simulink model "test_ENU"  (R2019b)
settings: Solver=VariableStepAuto  StartTime=0.0  StopTime=10.0  RelTol=1e-3
values from neighbouring files (symbols this model uses):
  own_height = 20000    [test_ENU_script.m]
  own_lat = 40    [test_ENU_script.m]
  own_long = 60    [test_ENU_script.m]
  traf_height = 15000    [test_ENU_script.m]
  traf_lat = 40    [test_ENU_script.m]
  traf_long = 60    [test_ENU_script.m]
settings Model: Creator=markwilkinson  LastModifiedBy=markwilkinson

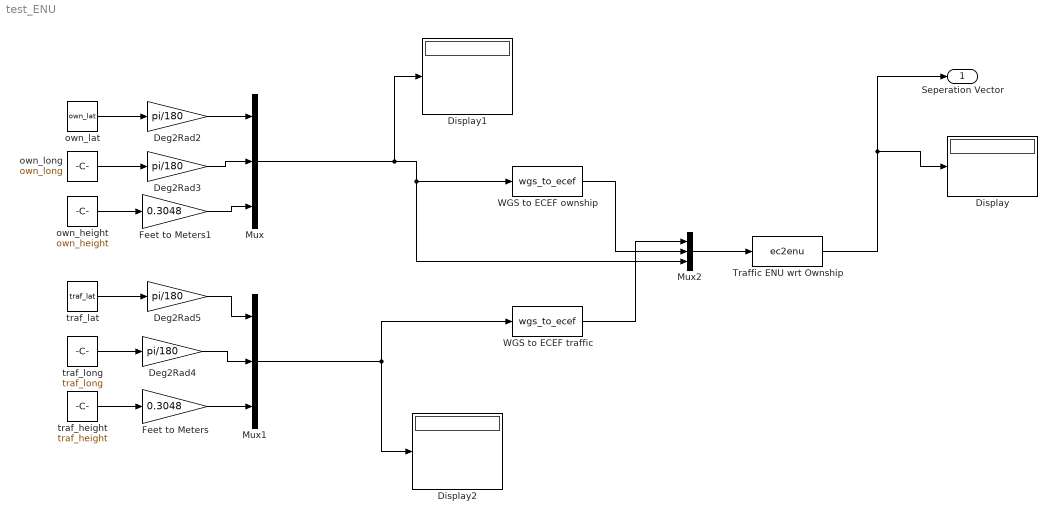
== system test_ENU ==
  Deg2Rad2 : Gain  RequirementInfo="{'other' 'cdf_srd - rev a.xlsx' '@Simulink_requirement_item_11' 'true' 'The system shall apply a gain of (pi/180) to the following inputs : - o_pos_lat - o_pos_lon - t_pos_lat - t_pos_lon  Commentary:Conversion from units of Degrees to Radians' '' } %GIDa_15e9ec68_b4a3_4827_8852_f140d8b86246"  Gain=pi/180
  Deg2Rad3 : Gain  RequirementInfo="{'other' 'cdf_srd - rev a.xlsx' '@Simulink_requirement_item_11' 'true' 'The system shall apply a gain of (pi/180) to the following inputs : - o_pos_lat - o_pos_lon - t_pos_lat - t_pos_lon  Commentary:Conversion from units of Degrees to Radians' '' } %GIDa_1b4d7c2c_606a_4deb_b429_1d850f30a73c"  Gain=pi/180
  Deg2Rad4 : Gain  RequirementInfo="{'other' 'cdf_srd - rev a.xlsx' '@Simulink_requirement_item_11' 'true' 'The system shall apply a gain of (pi/180) to the following inputs : - o_pos_lat - o_pos_lon - t_pos_lat - t_pos_lon  Commentary:Conversion from units of Degrees to Radians' '' } %GIDa_4a1cf90d_1327_49fa_91f0_70074aaa6b8f"  Gain=pi/180
  Deg2Rad5 : Gain  RequirementInfo="{'other' 'cdf_srd - rev a.xlsx' '@Simulink_requirement_item_11' 'true' 'The system shall apply a gain of (pi/180) to the following inputs : - o_pos_lat - o_pos_lon - t_pos_lat - t_pos_lon  Commentary:Conversion from units of Degrees to Radians' '' } %GIDa_68d829dd_f456_47fb_b7bd_7a116cacfa33"  Gain=pi/180
  Display : Display
  Display1 : Display
  Display2 : Display
  Feet to Meters : Gain  RequirementInfo="{'other' 'cdf_srd - rev a.xlsx' '@Simulink_requirement_item_12' 'true' 'The system shall apply a gain of 0.3048 to the following inputs : - o_pos_hgt - t_pos_hgt  Commentary:Conversion from units of feet to meters.' '' } %GIDa_1b2707cb_55ff_43b9_9ce0_0b6e1738a47f"  Gain=0.3048
  Feet to Meters1 : Gain  RequirementInfo="{'other' 'cdf_srd - rev a.xlsx' '@Simulink_requirement_item_12' 'true' 'The system shall apply a gain of 0.3048 to the following inputs : - o_pos_hgt - t_pos_hgt  Commentary:Conversion from units of feet to meters.' '' } %GIDa_73eaead6_38ef_47dd_a350_473f94a1f435"  Gain=0.3048
  Mux : Mux  RequirementInfo={} %GIDa_11867de4_8b9e_40eb_aa00_15ef062c16cf  Inputs=3
  Mux1 : Mux  RequirementInfo={} %GIDa_a07eb5ad_cb16_4cb2_8848_a4951b9d24eb  Inputs=3
  Mux2 : Mux  RequirementInfo={} %GIDa_dd87e64f_c0b1_4b86_a794_5fa7b9fe9044  Inputs=3
  Traffic ENU wrt Ownship : MATLABFcn  RequirementInfo={} %GIDa_8ac9cbbc_0c16_4e28_a971_ada722eea671  MATLABFcn=ec2enu
  WGS to ECEF ownship : MATLABFcn  RequirementInfo={} %GIDa_618d9f77_e347_4e22_8868_920bad7f9791  MATLABFcn=wgs_to_ecef
  WGS to ECEF traffic : MATLABFcn  RequirementInfo={} %GIDa_716f94d1_246d_45bd_97d9_09e47c4700e4  MATLABFcn=wgs_to_ecef
  own_height : Constant  Value=own_height
  own_lat : Constant  Value=own_lat
  own_long : Constant  Value=own_long
  traf_height : Constant  Value=traf_height
  traf_lat : Constant  Value=traf_lat
  traf_long : Constant  Value=traf_long
  Seperation Vector : Outport  RequirementInfo={} %GIDa_56ef3359_7248_4d0a_9d79_aaecc928cceb  SignalName=s_out
  wires:
  WGS to ECEF traffic/1 -> Mux2/1
  Mux/1 -> Display1/1, Mux2/3, WGS to ECEF ownship/1
  Mux1/1 -> Display2/1, WGS to ECEF traffic/1
  WGS to ECEF ownship/1 -> Mux2/2
  own_long/1 -> Deg2Rad3/1
  traf_long/1 -> Deg2Rad4/1
  Traffic ENU wrt Ownship/1 -> Seperation Vector/1, Display/1
  traf_height/1 -> Feet to Meters/1
  own_height/1 -> Feet to Meters1/1
  Mux2/1 -> Traffic ENU wrt Ownship/1
  traf_lat/1 -> Deg2Rad5/1
  own_lat/1 -> Deg2Rad2/1
  Feet to Meters/1 -> Mux1/3
  Feet to Meters1/1 -> Mux/3
  Deg2Rad2/1 -> Mux/1
  Deg2Rad3/1 -> Mux/2
  Deg2Rad4/1 -> Mux1/2
  Deg2Rad5/1 -> Mux1/1
